simulink model "ec_simple_trajectory"  (R2022a)
settings: Solver=ode3  StartTime=0.0  StopTime=inf  FixedStep=0.05  RelTol=1e-3
libraries: EcBlockToolbox x2

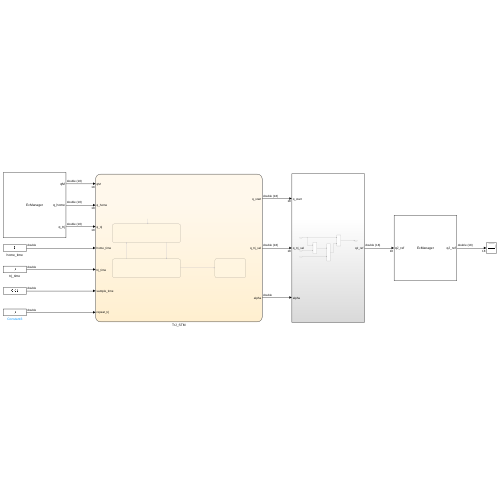
[thumbnail: Simulink's stored preview of the top-level diagram]
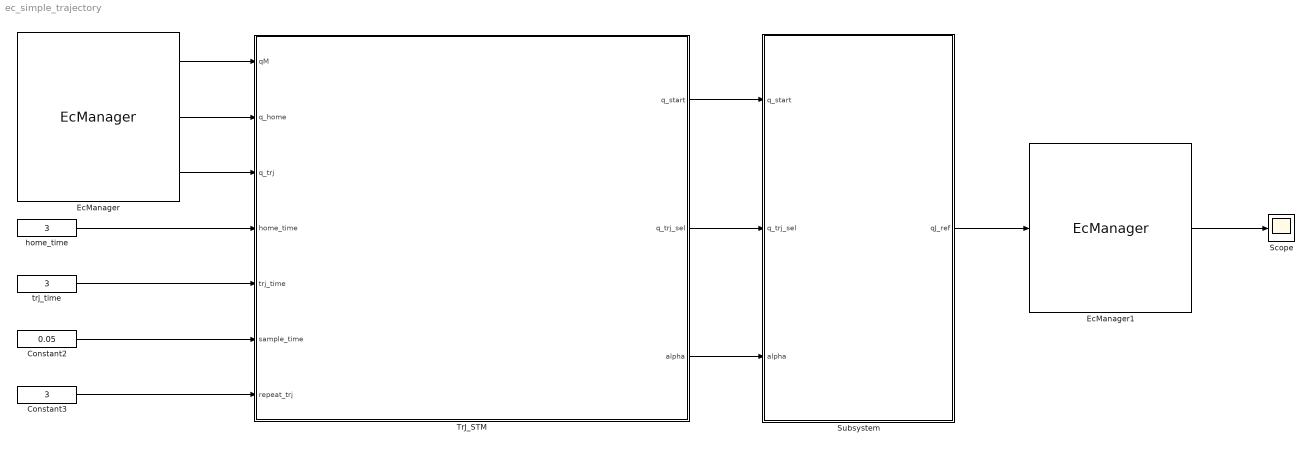
== system ec_simple_trajectory ==
  Constant2 : Constant  Value=0.05
  Constant3 : Constant  Value=3
  EcManager : EcBlockToolbox/EcManager  PowList={}  ReadingsList={'qM', 'q_home', 'q_trj'}  ReferencesList={}  ImuList={}  FtList={}
  EcManager1 : EcBlockToolbox/EcManager  PowList={}  ReadingsList={'qJ_ref'}  ReferencesList={'qJ_ref'}  ImuList={}  FtList={}
  Scope : Scope
  Subsystem : Subsystem
  TrJ_STM : Stateflow chart  TreatAsAtomicUnit=on
  home_time : Constant  Value=3
  trj_time : Constant  Value=3
  wires:
  home_time/1 -> TrJ_STM/4(home_time)
  trj_time/1 -> TrJ_STM/5(trj_time)
  Constant2/1 -> TrJ_STM/6(sample_time)
  Constant3/1 -> TrJ_STM/7(repeat_trj)
  TrJ_STM/1(q_start) -> Subsystem/1(q_start)
  TrJ_STM/2(q_trj_sel) -> Subsystem/2(q_trj_sel)
  TrJ_STM/3(alpha) -> Subsystem/3(alpha)
  Subsystem/1(qJ_ref) -> EcManager1/1
  EcManager1/1 -> Scope/1
  EcManager/1 -> TrJ_STM/1(qM)
  EcManager/2 -> TrJ_STM/2(q_home)
  EcManager/3 -> TrJ_STM/3(q_trj)

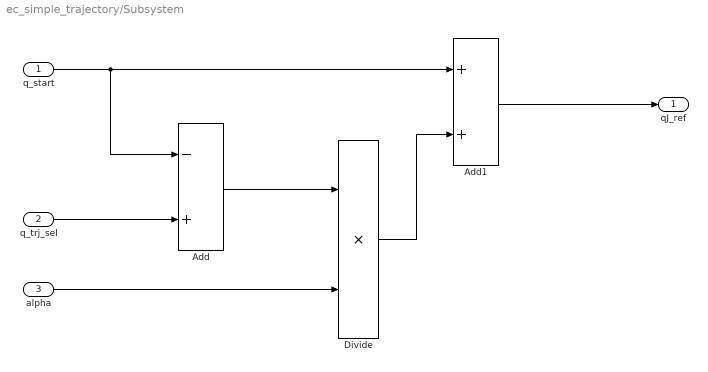
== system ec_simple_trajectory/Subsystem ==
  q_start : Inport
  q_trj_sel : Inport  Port=2
  alpha : Inport  Port=3
  Add : Sum  Inputs=-+
  Add1 : Sum
  Divide : Product  Inputs=**
  qJ_ref : Outport
  wires:
  Divide/1 -> Add1/2
  Add/1 -> Divide/1
  q_start/1 -> Add1/1, Add/1
  q_trj_sel/1 -> Add/2
  alpha/1 -> Divide/2
  Add1/1 -> qJ_ref/1

== stateflow chart ec_simple_trajectory/TrJ_STM ==
  state Homing
    en: q_trj_sel = q_home; time=0;alpha=0;
    du: time=time + sample_time;
    tau=time/home_time;
    alpha = ((6*tau - 15)*tau + 10)*tau*tau*tau;
  state Stop
    en: alpha=0;
  state Trajectory
    en: q_trj_sel = q_trj; time=0;alpha=0;
    du: time=time + sample_time;
    tau=time/home_time;
    alpha = ((6*tau - 15)*tau + 10)*tau*tau*tau;
  (default) -> Homing : /{q_start=qM;}
  Trajectory -> Homing [order 1] : [time >= trj_time]/{q_start = q_trj;}
  Homing -> Trajectory : [time >= home_time]/{trj_rep_count=trj_rep_count+1; q_start = q_home;}
  Trajectory -> Stop [order 2] : [trj_rep_count == repeat_trj]
  data: q_start output; qM input; q_home input; q_trj input; q_trj_sel output; home_time input; trj_time input; sample_time input; repeat_trj input; time local =0; trj_rep_count local =0; alpha output; tau local =0
